simulink model "ch53_sim_compat"  (R2012a)
settings: Solver=ode45  SolverMode=SingleTasking  StartTime=0.0  StopTime=40  RelTol=1e-3
undefined symbols (not defined in the file): A, althold, B, C, collective_dist, compensator, cyclic_dist, D, h_wish, K, q_initial, q_wish, sigbuilder_block, surge, thetaf_initial, thetaf_wish, u_initial, u_wish, w_initial, w_wish
libraries: simulink_extras x5, simulink x2
settings Model: CovMetricSettings=dwe  CovHtmlReporting=off  covSaveCumulativeToWorkspaceVar=off  CovSaveSingleToWorkspaceVar=off  CovExternalEMLEnable=on  Creator=KILKISZenbook  LastModifiedBy=KILKISZenbook
settings DataIOCC: SaveFormat=Structure  SaveOutput=off  SaveState=on  ReturnWorkspaceOutputs=off  OutputSaveName=sim.yout
settings OptimizationCC: LifeSpan=inf  SimCompilerOptimization=Off
settings DebuggingCC: FcnCallInpInsideContextMsg=Enable All
settings HardwareCC: ProdWordSize=32  ProdHWDeviceType=Specified
settings SFSimCC: SimUseLocalCustomCode=off
settings RTWCC: RTWUseLocalCustomCode=off  RTWCompilerOptimization=Off
settings GRTTargetCC: CodeReplacementLibrary=C99 (ISO)  CPPClassGenCompliant=off

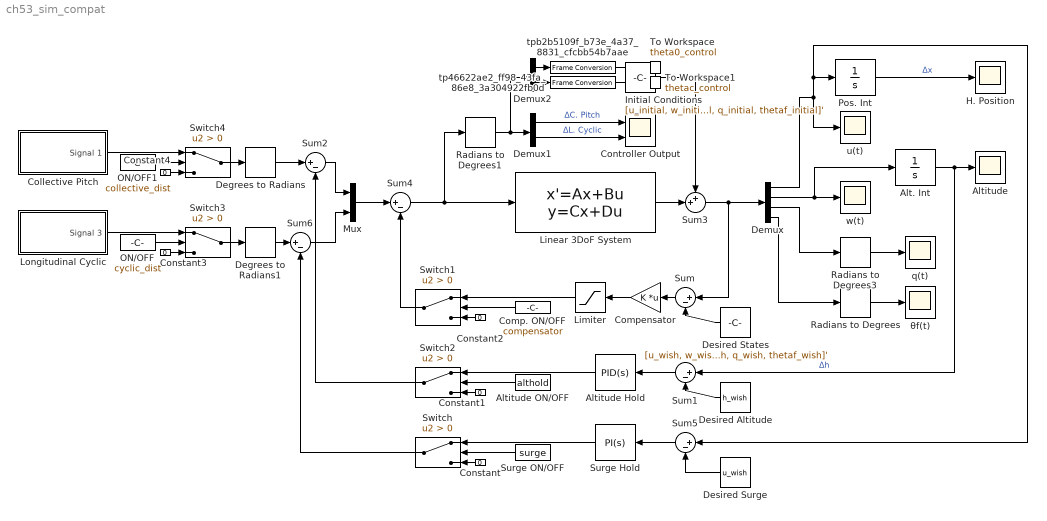
== system ch53_sim_compat ==
  Alt. Int : TransferFcn  Denominator=[1 0]
  Altitude : Scope
      settings: TimeRange=auto  MaxDataPoints=5000  SaveToWorkspace=off  SaveName=ScopeData2  YMin=-0.00273  YMax=0.0099  SampleTime=-1
  Altitude Hold : simulink/Continuous/PID Controller  Controller=PID  TimeDomain=Continuous-time  SampleTime=-1  IntegratorMethod=Forward Euler  FilterMethod=Forward Euler  Form=Parallel  UseFilter=on  ControllerParametersSource=internal  P=-0.890521666305557  I=-0.214571197732449  D=-0.379646995986737  N=3560.86236447433  InitialConditionSource=internal  InitialConditionForIntegrator=0  InitialConditionForFilter=0  ExternalReset=none  LimitOutput=off  UpperSaturationLimit=inf  LowerSaturationLimit=-inf  LinearizeAsGain=on  AntiWindupMode=none  Kb=1  TrackingMode=off  Kt=1  PParamMin=[]  PParamMax=[]  IParamMin=[]  IParamMax=[]  DParamMin=[]  DParamMax=[]  NParamMin=[]  NParamMax=[]  KbParamMin=[]  KbParamMax=[]  KtParamMin=[]  KtParamMax=[]  POutMin=[]  POutMax=[]  IOutMin=[]  IOutMax=[]  DOutMin=[]  DOutMax=[]  NOutMin=[]  NOutMax=[]  KbOutMin=[]  KbOutMax=[]  KtOutMin=[]  KtOutMax=[]  IntegratorOutMin=[]  IntegratorOutMax=[]  FilterOutMin=[]  FilterOutMax=[]  SumOutMin=[]  SumOutMax=[]  SumI1OutMin=[]  SumI1OutMax=[]  SumI2OutMin=[]  SumI2OutMax=[]  SumI3OutMin=[]  SumI3OutMax=[]  SumDOutMin=[]  SumDOutMax=[]  SaturationOutMin=[]  SaturationOutMax=[]  IntegratorContinuousStateAttributes=''  IntegratorStateMustResolveToSignalObject=off  IntegratorRTWStateStorageClass=Auto  FilterContinuousStateAttributes=''  FilterStateMustResolveToSignalObject=off  FilterRTWStateStorageClass=Auto  DifferentiatorICPrevScaledInput=0  DifferentiatorOutMin=[]  DifferentiatorOutMax=[]
  Altitude ON/OFF : Constant  Value=althold  VectorParams1D=off
  Collective Pitch : Subsystem  Tag=STV Subsys  LoadFcn=sigbuilder_block('load');  StartFcn=sigbuilder_block('start');  StopFcn=sigbuilder_block('stop');  ClipboardFcn=sigbuilder_block('clipboard');  mask(Sigbuilder block){tuvar=[0:10]}
      mask help: Simulink:masks:SigbuilderBlock_MD
      mask init:
      | if ~strcmp(get_param(bdroot(gcbh),'SimulationStatus'),'stopped') tuvar = sigbuilder_block('maskInit'); end
      settings: CopyFcn=sigbuilder_block('copy');  DeleteFcn=sigbuilder_block('delete');  ModelCloseFcn=sigbuilder_block('modelClose');  PreSaveFcn=sigbuilder_block('preSave');  PauseFcn=sigbuilder_block('pause');  ContinueFcn=sigbuilder_block('continue');  NameChangeFcn=sigbuilder_block('namechange');  OpenFcn=sigbuilder_block('open',[543.75 233.25 550.5 399.75 ]);  CloseFcn=sigbuilder_block('close');
      mask Display: plot(0, 0, 100, 100,[2, 2, 32, 32, 2], [68, 8, 8, 68, 68],[32, 2], [38, 38], [32, 19, 2],[53, 60, 44], [32, 17, 17, 2],[16, 16, 31, 31]);txt = getActiveGroup(gcbh);text(2, 100, txt,'verticalAlignment', 'top');
  Comp. ON/OFF : Constant  Value=compensator  VectorParams1D=off
  Compensator : Gain  Gain=K  Multiplication=Matrix(K*u)
  Constant{,1..4} (5 alike) : Constant  Value=0
  Controller Output : Scope  NumInputPorts=2
      settings: TimeRange=auto  ShowLegends=on  MaxDataPoints=5000  SaveToWorkspace=off  YMin=-13.30156~-5  YMax=5.51935~5  SampleTime=-1
  Degrees to Radians : simulink_extras/Transformations/Degrees to Radians
  Degrees to Radians1 : simulink_extras/Transformations/Degrees to Radians
  Demux : Demux
  Demux1 : Demux  Outputs=2
  Demux2 : Demux  Outputs=2
  Desired Altitude : Constant  Value=h_wish
  Desired States : Constant  Value=[u_wish, w_wish, q_wish, thetaf_wish]'  VectorParams1D=off
  "Desired Surge " : Constant  Value=u_wish
  H. Position : Scope
      settings: TimeRange=auto  MaxDataPoints=5000  SaveToWorkspace=off  YMin=-1.31401  YMax=11.82607  SampleTime=-1
  Initial Conditions : Constant  Value=[u_initial, w_initial, q_initial, thetaf_initial]'
  Limiter : Saturate  UpperLimit=0.174533  LowerLimit=-0.174533
  Linear 3DoF System : StateSpace  A=A  B=B  C=C  D=D  X0=[]  ContinuousStateAttributes='state_matrix'
  Longitudinal Cyclic : Subsystem  Tag=STV Subsys  LoadFcn=sigbuilder_block('load');  StartFcn=sigbuilder_block('start');  StopFcn=sigbuilder_block('stop');  ClipboardFcn=sigbuilder_block('clipboard');  mask(Sigbuilder block){tuvar=[0:10]}
      mask help: Simulink:masks:SigbuilderBlock_MD
      mask init:
      | if ~strcmp(get_param(bdroot(gcbh),'SimulationStatus'),'stopped') tuvar = sigbuilder_block('maskInit'); end
      settings: CopyFcn=sigbuilder_block('copy');  DeleteFcn=sigbuilder_block('delete');  ModelCloseFcn=sigbuilder_block('modelClose');  PreSaveFcn=sigbuilder_block('preSave');  PauseFcn=sigbuilder_block('pause');  ContinueFcn=sigbuilder_block('continue');  NameChangeFcn=sigbuilder_block('namechange');  OpenFcn=sigbuilder_block('open',[480 165.75 551.25 400.5 ]);  CloseFcn=sigbuilder_block('close');
      mask Display: plot(0, 0, 100, 100,[2, 2, 32, 32, 2], [68, 8, 8, 68, 68],[32, 2], [38, 38], [32, 19, 2],[53, 60, 44], [32, 17, 17, 2],[16, 16, 31, 31]);txt = getActiveGroup(gcbh);text(2, 100, txt,'verticalAlignment', 'top');
  Mux : Mux  Inputs=2
  ON/OFF : Constant  Value=cyclic_dist  VectorParams1D=off
  ON/OFF1 : Constant  Value=collective_dist  VectorParams1D=off
  Pos. Int : TransferFcn  Denominator=[1 0]
  Radians to Degrees : simulink_extras/Transformations/Radians to Degrees
  Radians to Degrees1 : simulink_extras/Transformations/Radians to Degrees
  Radians to Degrees3 : simulink_extras/Transformations/Radians to Degrees
  Sum{,1..2,4..6} (6 alike) : Sum  Inputs=|+-
  Sum3 : Sum  Inputs=++|
  Surge Hold : simulink/Continuous/PID Controller  Controller=PI  TimeDomain=Continuous-time  SampleTime=-1  IntegratorMethod=Forward Euler  FilterMethod=Forward Euler  Form=Parallel  UseFilter=on  ControllerParametersSource=internal  P=0.00455207149246213  I=0.00631604464079722  D=0  N=100  InitialConditionSource=internal  InitialConditionForIntegrator=0  InitialConditionForFilter=0  ExternalReset=none  LimitOutput=off  UpperSaturationLimit=inf  LowerSaturationLimit=-inf  LinearizeAsGain=on  AntiWindupMode=none  Kb=1  TrackingMode=off  Kt=1  PParamMin=[]  PParamMax=[]  IParamMin=[]  IParamMax=[]  DParamMin=[]  DParamMax=[]  NParamMin=[]  NParamMax=[]  KbParamMin=[]  KbParamMax=[]  KtParamMin=[]  KtParamMax=[]  POutMin=[]  POutMax=[]  IOutMin=[]  IOutMax=[]  DOutMin=[]  DOutMax=[]  NOutMin=[]  NOutMax=[]  KbOutMin=[]  KbOutMax=[]  KtOutMin=[]  KtOutMax=[]  IntegratorOutMin=[]  IntegratorOutMax=[]  FilterOutMin=[]  FilterOutMax=[]  SumOutMin=[]  SumOutMax=[]  SumI1OutMin=[]  SumI1OutMax=[]  SumI2OutMin=[]  SumI2OutMax=[]  SumI3OutMin=[]  SumI3OutMax=[]  SumDOutMin=[]  SumDOutMax=[]  SaturationOutMin=[]  SaturationOutMax=[]  IntegratorContinuousStateAttributes=''  IntegratorStateMustResolveToSignalObject=off  IntegratorRTWStateStorageClass=Auto  FilterContinuousStateAttributes=''  FilterStateMustResolveToSignalObject=off  FilterRTWStateStorageClass=Auto  DifferentiatorICPrevScaledInput=0  DifferentiatorOutMin=[]  DifferentiatorOutMax=[]
  Surge ON/OFF : Constant  Value=surge  VectorParams1D=off
  Switch{,1..4} (5 alike) : Switch  Criteria=u2 > Threshold
  To Workspace : ToWorkspace  VariableName=theta0_control  SampleTime=-1
  To Workspace1 : ToWorkspace  VariableName=thetac_control  SampleTime=-1
  q(t) : Scope
      settings: TimeRange=auto  MaxDataPoints=5000  SaveToWorkspace=off  SaveName=ScopeData2  YMin=-7.56155  YMax=9.58563  SampleTime=-1
  tp46622ae2_ff98_43fa_86e8_3a304922fb0d : FrameConversion
  tpb2b5109f_b73e_4a37_8831_cfcbb54b7aae : FrameConversion
  u(t) : Scope
      settings: TimeRange=auto  MaxDataPoints=5000  SaveToWorkspace=off  SaveName=ScopeData  YMin=-3.28446  YMax=6.08098  SampleTime=-1
  w(t) : Scope
      settings: TimeRange=auto  MaxDataPoints=5000  SaveToWorkspace=off  YMin=-0.01108  YMax=0.01096  SampleTime=-1
  θf(t) : Scope
      settings: TimeRange=auto  MaxDataPoints=5000  SaveToWorkspace=off  SaveName=ScopeData3  YMin=-7.77975  YMax=16.00838  SampleTime=-1
  wires:
  Radians to Degrees/1 -> θf(t)/1
  Alt. Int/1 -> Sum1/1, Altitude/1  "Δh"
  Demux/3 -> Radians to Degrees3/1
  Radians to Degrees3/1 -> q(t)/1
  Pos. Int/1 -> H. Position/1  "Δx"
  Compensator/1 -> Limiter/1
  Demux/4 -> Radians to Degrees/1
  Demux1/1 -> Controller Output/1  "ΔC. Pitch"
  Demux1/2 -> Controller Output/2  "ΔL. Cyclic"
  Radians to Degrees1/1 -> Demux2/1, Demux1/1
  Demux/1 -> Sum5/1, Pos. Int/1, u(t)/1
  Degrees to Radians/1 -> Sum2/1
  Sum/1 -> Compensator/1
  Desired States/1 -> Sum/2
  Desired Altitude/1 -> Sum1/2
  Sum1/1 -> Altitude Hold/1
  Sum3/1 -> Sum/1, Demux/1
  Linear 3DoF System/1 -> Sum3/2
  Demux/2 -> Alt. Int/1, w(t)/1
  Initial Conditions/1 -> Sum3/1
  "Desired Surge "/1 -> Sum5/2
  Sum5/1 -> Surge Hold/1
  Surge Hold/1 -> Switch/1
  Surge ON/OFF/1 -> Switch/2
  Limiter/1 -> Switch1/1
  Switch1/1 -> Sum4/2
  Comp. ON/OFF/1 -> Switch1/2
  Altitude ON/OFF/1 -> Switch2/2
  Altitude Hold/1 -> Switch2/1
  Constant/1 -> Switch/3
  Constant1/1 -> Switch2/3
  Constant2/1 -> Switch1/3
  Sum6/1 -> Mux/2
  Sum2/1 -> Mux/1
  Sum4/1 -> Radians to Degrees1/1, Linear 3DoF System/1
  Mux/1 -> Sum4/1
  Longitudinal Cyclic/1(Signal 3) -> Switch3/1
  Switch3/1 -> Degrees to Radians1/1
  ON/OFF/1 -> Switch3/2
  Constant3/1 -> Switch3/3
  ON/OFF1/1 -> Switch4/2
  Constant4/1 -> Switch4/3
  Collective Pitch/1(Signal 1) -> Switch4/1
  Switch4/1 -> Degrees to Radians/1
  Degrees to Radians1/1 -> Sum6/1
  Switch2/1 -> Sum2/2
  Switch/1 -> Sum6/2
  Demux2/1 -> tpb2b5109f_b73e_4a37_8831_cfcbb54b7aae/1
  tpb2b5109f_b73e_4a37_8831_cfcbb54b7aae/1 -> To Workspace/1
  Demux2/2 -> tp46622ae2_ff98_43fa_86e8_3a304922fb0d/1
  tp46622ae2_ff98_43fa_86e8_3a304922fb0d/1 -> To Workspace1/1

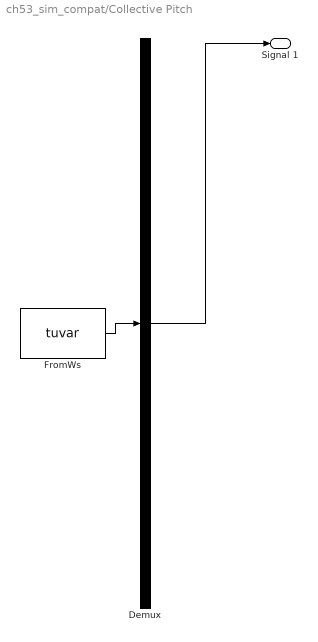
== system ch53_sim_compat/Collective Pitch ==
  Demux : Demux  Tag=STV Demux  Outputs=1
  FromWs : FromWorkspace  Tag=STV FromWs  VariableName=tuvar  SampleTime=0
      SigBuilderData=|
      | common.afterFinalStr = 'Extrapolate'
      | common.sampleTime = 0
      | dataSet.timeRange = [0 10]
      | dataSet.name = 'Manual Inputs'
      | sbobj.Groups.Name = 'Manual Inputs'
      | sbobj.Groups.Signals.Name = 'Signal 1'
      | sbobj.Groups.Signals.XData = [0 0.5 1 10]
      | sbobj.Groups.Signals.YData = [0 0 0 0]
  Signal 1 : Outport  Tag=STV Outport
  wires:
  Demux/1 -> Signal 1/1
  FromWs/1 -> Demux/1

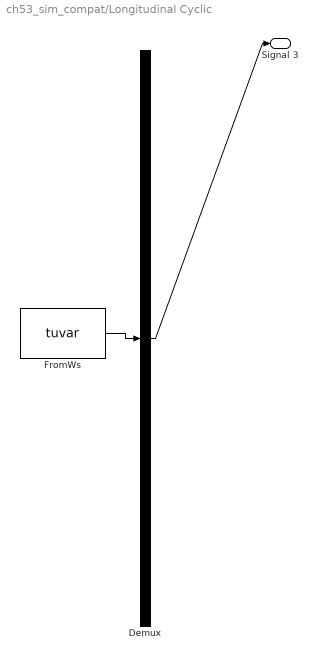
== system ch53_sim_compat/Longitudinal Cyclic ==
  Demux : Demux  Tag=STV Demux  Outputs=1
  FromWs : FromWorkspace  Tag=STV FromWs  VariableName=tuvar  SampleTime=0
      SigBuilderData=|
      | common.afterFinalStr = 'Extrapolate'
      | common.sampleTime = 0
      | dataSet.timeRange = [0 10]
      | dataSet.name = 'Manual Inputs'
      | sbobj.Groups.Name = 'Manual Inputs'
      | sbobj.Groups.Signals.Name = 'Signal 3'
      | sbobj.Groups.Signals.XData = [0 0.5 0.5 1 1 10]
      | sbobj.Groups.Signals.YData = [0 0 -1 -1 0 0]
  Signal 3 : Outport  Tag=STV Outport
  wires:
  FromWs/1 -> Demux/1
  Demux/1 -> Signal 3/1
